simulink model "Resonator16_order_FIR"  (R2019a)
settings: Solver=FixedStepDiscrete  StartTime=0.0  StopTime=10  FixedStep=0.001  RelTol=1e-3
libraries: dspxfrm3 x2, simulink x1
settings Model: Creator=vardhah  LastModifiedBy=vardhah
settings DataIOCC: ReturnWorkspaceOutputs=off
settings DebuggingCC: ArithmeticOperatorsInVariantConditions=warning

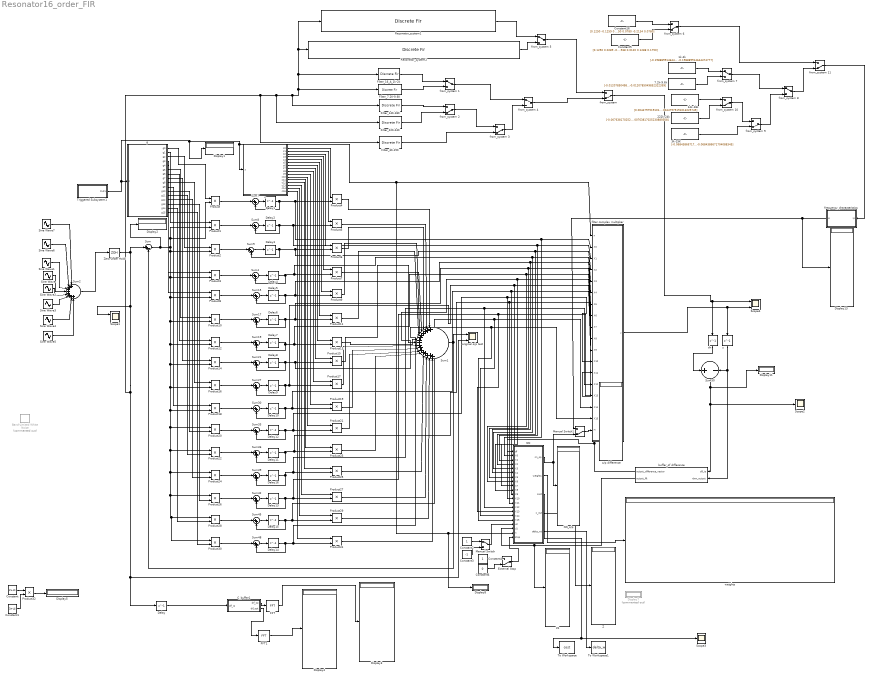
== system Resonator16_order_FIR ==
  "14k-18k " : Constant  Value=[0.00447975191013225745 0.0111493911810838543 0.0275893297063002849 -0.183954681451905411 0.0755136163583744469 0.0976817056268990125 -0.238475271342986128 0.121471156344241021 0.121471156344241021 -0.238475271342986128 0.0976817056268990125 0.0755136163583744469 -0.183954681451905411 0.0275893297063002849 0.0111493911810838543 0.00447975191013225745]  VectorParams1D=off
  1k-2k : Constant  Value=[-0.198889914644374777 0.0882189428518377339 0.0736891495871065116 0.0638368801789635787 0.0566372642221577294 0.0523172683654103132 0.0494565343907736044 0.048157521822162791 0.048157521822162791 0.0494565343907736044 0.0523172683654103132 0.0566372642221577294 0.0638368801789635787 0.0736891495871065116 0.0882189428518377339 -0.198889914644374777]  VectorParams1D=off
  222k-24k : Constant  Value=[-0.00763817025230889308 0.108944026972857946 -0.0989847012675625776 0.124240247797868963 -0.129657713018954679 0.114438069344974691 -0.0787108015776764036 0.0280491419731783154 0.0280491419731783154 -0.0787108015776764036 0.114438069344974691 -0.129657713018954679 0.124240247797868963 -0.0989847012675625776 0.108944026972857946 -0.00763817025230889308]  VectorParams1D=off
  3k-15K : Constant  Value=[-0.0684386671704088345 -0.0216035519389094557 -0.0869907772510868094 -0.0695372998678755599 0.0160068430386171648 -0.171506412844009415 -0.104404398490726372 0.48413102780480427 0.48413102780480427 -0.104404398490726372 -0.171506412844009415 0.0160068430386171648 -0.0695372998678755599 -0.0869907772510868094 -0.0216035519389094557 -0.0684386671704088345]  VectorParams1D=off
  "7.2k-9.6k " : Constant  Value=[-0.0120785049852322399 -0.0942455273574688279 0.0101245004695954266 0.125460404555770566 0.034165372769331126 -0.1614987160724079 -0.0984930555982914957 0.150982315564688691 0.150982315564688691 -0.0984930555982914957 -0.1614987160724079 0.034165372769331126 0.125460404555770566 0.0101245004695954266 -0.0942455273574688279 -0.0120785049852322399]  VectorParams1D=off
  Band-Limited White Noise : simulink/Sources/Band-Limited White Noise  Commented=on  Cov=[0.5]  Ts=0.000003  seed=[23341]
  C_buffer1 : MATLAB Function  TreatAsAtomicUnit=on
  Constant : Constant  Value=2+3i
  Constant1 : Constant  Value=3+4i
  Constant16 : Constant  Value=[0.1250 -0.1259 0 0.0375 0 0.0104 -0.0366 0.0104 0 0.0375 0 -0.1259 0.1250 0.0780 -0.2134 0.0780]  VectorParams1D=off
  Constant2 : Constant
  Constant3 : Constant  Value=-1
  Constant4 : Constant
  Constant5 : Constant  Value=[0.1250 0.0289 -0.0404 -0.0525 -0.0313 -0.0120 -0.0038 0.0018 0 -0.0289 -0.0846 -0.1243 -0.0938 0.0120 0.1288 0.1750]  VectorParams1D=off
  Constant6 : Constant  Value=0
  Delay{,1..16} (17 alike) : Delay  DelayLength=1  InitialCondition=0
  Display{1..5,8,11,13} (8 alike) : Display
  Display7 : Display  Commented=on
  External Stop : ManualSwitch  CurrentSetting=0
  FFT : dspxfrm3/FFT  FFTImplementation=Auto  CompMethod=Table lookup  TableOpt=NEW  TableOptActive=Speed  BitRevOrder=off  Normalize=on  InheritFFTLength=on  FFTLength=64  WrapInput=on  roundingMode=Floor  overflowMode=off  firstCoeffDataTypeStr=Inherit: Same word length as input  firstCoeffLastDataTypeStr=Inherit: Same word length as input  outputMin=[]  outputMax=[]
  FFT1 : dspxfrm3/FFT  FFTImplementation=Auto  CompMethod=Table lookup  TableOpt=NEW  TableOptActive=Speed  BitRevOrder=off  Normalize=on  InheritFFTLength=on  FFTLength=64  WrapInput=on  roundingMode=Floor  overflowMode=off  firstCoeffDataTypeStr=Inherit: Same word length as input  firstCoeffLastDataTypeStr=Inherit: Same word length as input  outputMin=[]  outputMax=[]
  Filter_14K-18K : DiscreteFir  Tag=BlockMethodSubSystem  Coefficients=[0.00447975191013225745 0.0111493911810838543 0.0275893297063002849 -0.183954681451905411 0.0755136163583744469 0.0976817056268990125 -0.238475271342986128 0.121471156344241021 0.121471156344241021 -0.238475271342986128 0.0976817056268990125 0.0755136163583744469 -0.183954681451905411 0.0275893297063002849 0.0111493911810838543 0.00447975191013225745]  InputProcessing=Columns as channels (frame based)
  Filter_16_A_1k-2k : DiscreteFir  Tag=BlockMethodSubSystem  Coefficients=[-0.198889914644374777 0.0882189428518377339 0.0736891495871065116 0.0638368801789635787 0.0566372642221577294 0.0523172683654103132 0.0494565343907736044 0.048157521822162791 0.048157521822162791 0.0494565343907736044 0.0523172683654103132 0.0566372642221577294 0.0638368801789635787 0.0736891495871065116 0.0882189428518377339 -0.198889914644374777]  InputProcessing=Columns as channels (frame based)
  Filter_22K-24K : DiscreteFir  Tag=BlockMethodSubSystem  Coefficients=[-0.00763817025230889308 0.108944026972857946 -0.0989847012675625776 0.124240247797868963 -0.129657713018954679 0.114438069344974691 -0.0787108015776764036 0.0280491419731783154 0.0280491419731783154 -0.0787108015776764036 0.114438069344974691 -0.129657713018954679 0.124240247797868963 -0.0989847012675625776 0.108944026972857946 -0.00763817025230889308]  InputProcessing=Columns as channels (frame based)
  Filter_3K-15K : DiscreteFir  Tag=BlockMethodSubSystem  Coefficients=[-0.0684386671704088345 -0.0216035519389094557 -0.0869907772510868094 -0.0695372998678755599 0.0160068430386171648 -0.171506412844009415 -0.104404398490726372 0.48413102780480427 0.48413102780480427 -0.104404398490726372 -0.171506412844009415 0.0160068430386171648 -0.0695372998678755599 -0.0869907772510868094 -0.0216035519389094557 -0.0684386671704088345]  InputProcessing=Columns as channels (frame based)
  "Filter_7.2K-9.6K " : DiscreteFir  Tag=BlockMethodSubSystem  Coefficients=[-0.0120785049852322399 -0.0942455273574688279 0.0101245004695954266 0.125460404555770566 0.034165372769331126 -0.1614987160724079 -0.0984930555982914957 0.150982315564688691 0.150982315564688691 -0.0984930555982914957 -0.1614987160724079 0.034165372769331126 0.125460404555770566 0.0101245004695954266 -0.0942455273574688279 -0.0120785049852322399]  InputProcessing=Columns as channels (frame based)
  Manual Switch : ManualSwitch
  Manual Switch1 : ManualSwitch  CurrentSetting=0  varsize=on
  NN : MATLAB Function  TreatAsAtomicUnit=on
  NN_o/p : Display
  Product{,1..32} (33 alike) : Product
  "Rezonator_system1 " : DiscreteFir  Tag=BlockMethodSubSystem  Coefficients=[0.1250 -0.1259 0 0.0375 0 0.0104 -0.0366 0.0104 0 0.0375 0 -0.1259 0.1250 0.0780 -0.2134 0.0780]  InputProcessing=Columns as channels (frame based)
  Rezonator_system2 : DiscreteFir  Tag=BlockMethodSubSystem  Coefficients=[0.1250 0.0289 -0.0404 -0.0525 -0.0313 -0.0120 -0.0038 0.0018 0 -0.0289 -0.0846 -0.1243 -0.0938 0.0120 0.1288 0.1750]  InputProcessing=Columns as channels (frame based)
  Scope1 : Scope  NumInputPorts=2
  Scope2 : Scope
  Scope3 : Scope
  Scope4 : Scope  NumInputPorts=2
  Sine Wave : Sin  Amplitude=0  Frequency=5000  SampleTime=0
  Sine Wave1 : Sin  Amplitude=0  Frequency=7000  SampleTime=0
  Sine Wave2 : Sin  Amplitude=0  Frequency=2000  SampleTime=0
  Sine Wave3 : Sin  Amplitude=0  Frequency=479  SampleTime=0
  Sine Wave4 : Sin  Amplitude=0  Frequency=100  SampleTime=0
  Sine Wave5 : Sin  Amplitude=3  Frequency=50  SampleTime=0
  Sine Wave6 : Sin  Amplitude=0  Frequency=11000  SampleTime=0
  Sine Wave7 : Sin  Amplitude=0  Frequency=17000  SampleTime=0
  Sum : Sum  Inputs=|+-
  Sum1 : Sum  Inputs=|++++++++++++++++
  Sum{4,7..9,15,17,19,21,27,30,33,36,39,42,45,48} (16 alike) : Sum  Inputs=|++
  Sum2 : Sum  Inputs=|++++++++
  Sum50 : Sum  Inputs=+-
  To Workspace : ToWorkspace  VariableName=cost  SampleTime=-1
      settings: Save2DSignal=2-D array (concatenate along first dimension)
  To Workspace1 : ToWorkspace  VariableName=delta_w  SampleTime=-1
      settings: Save2DSignal=2-D array (concatenate along first dimension)
  Triggered Subsystem1 : Subsystem  TreatAsAtomicUnit=on
  Z : Display
  Z1 : Display
  Zero-Order Hold : ZeroOrderHold  SampleTime=0.001
  buffer_of difference : MATLAB Function  TreatAsAtomicUnit=on
  c : MATLAB Function  TreatAsAtomicUnit=on
  dn : Delay  DelayLength=1  InitialCondition=0
  filter complex multiplier : MATLAB Function  TreatAsAtomicUnit=on
  frequency_characteristics : MATLAB Function  TreatAsAtomicUnit=on
  from_system {,2..3,6,9..11} (7 alike) : ManualSwitch  CurrentSetting=0
  from_system {1,4..5,7..8} (5 alike) : ManualSwitch
  g : MATLAB Function  TreatAsAtomicUnit=on
  o/p difference : Display
  "original o/p test " : Scope  NumInputPorts=2
  weights : Display
  y : Delay  DelayLength=1  InitialCondition=0
  wires:
  Delay1/1 -> filter complex multiplier/2(X0), NN/2(X0), Product4/2, Sum7/2
  c/1(c0) -> Product4/1
  c/2(c1) -> Product5/1
  c/3(c2) -> Product6/1
  c/4(c3) -> Product7/1
  Delay2/1 -> Sum8/2, filter complex multiplier/3(X1), NN/3(X1), Product5/2
  Delay3/1 -> NN/4(X2), filter complex multiplier/4(X2), Product6/2, Sum9/2
  Delay4/1 -> Sum4/2, NN/5(X3), filter complex multiplier/5(X3), Product7/2
  Sum1/1 -> "original o/p test "/1, Sum/2
  g/1(g0) -> Product/1
  g/2(g1) -> Product1/1
  g/3(g2) -> Product2/1
  g/4(g3) -> Product3/1
  Sum4/1 -> Delay4/1
  Sum9/1 -> Delay3/1
  Sum8/1 -> Delay2/1
  Sum7/1 -> Delay1/1
  Product4/1 -> Sum1/1
  Product5/1 -> Sum1/2
  Product6/1 -> Sum1/3
  Product7/1 -> Sum1/4
  Triggered Subsystem1/1(Out1) -> Display1/1, c/1(n), Display8/1, NN/20(n), filter complex multiplier/1(n), g/1(n)
  Sum/1 -> Display2/1, Product1/2, Product/2, Product2/2, Product10/2, Product12/2, Product14/2, Product16/2, Product30/1, Product28/1, Product26/1, Product24/1, Product22/1, Product20/1, Product18/2, Product8/2, Product3/2
  Product3/1 -> Sum4/1
  Product2/1 -> Sum9/1
  Product1/1 -> Sum8/1
  Product/1 -> Sum7/1
  Product8/1 -> Sum15/1
  Sum15/1 -> Delay5/1
  Delay5/1 -> filter complex multiplier/6(X4), NN/6(X4), Product9/2, Sum15/2
  Product10/1 -> Sum17/1
  Sum17/1 -> Delay6/1
  Delay6/1 -> filter complex multiplier/7(X5), NN/7(X5), Product11/2, Sum17/2
  Product12/1 -> Sum19/1
  Sum19/1 -> Delay7/1
  Delay7/1 -> filter complex multiplier/8(X6), NN/8(X6), Product13/2, Sum19/2
  Product14/1 -> Sum21/1
  Sum21/1 -> Delay8/1
  Delay8/1 -> filter complex multiplier/9(X7), NN/9(X7), Product15/2, Sum21/2
  g/5(g4) -> Product8/1
  g/6(g5) -> Product10/1
  g/7(g6) -> Product12/1
  g/8(g7) -> Product14/1
  c/5(c4) -> Product9/1
  c/6(c5) -> Product11/1
  c/7(c6) -> Product13/1
  c/8(c7) -> Product15/1
  Product9/1 -> Sum1/5
  Product11/1 -> Sum1/6
  Product13/1 -> Sum1/7
  Product15/1 -> Sum1/8
  Product16/1 -> Sum27/1
  Sum27/1 -> Delay9/1
  Delay9/1 -> Product17/2, filter complex multiplier/10(X8), NN/10(X8), Sum27/2
  Sum30/1 -> Delay10/1
  Delay10/1 -> filter complex multiplier/11(X9), NN/11(X9), Product19/2, Sum30/2
  Product18/1 -> Sum30/1
  Sum33/1 -> Delay12/1
  Delay12/1 -> NN/12(X10), filter complex multiplier/12(X10), Product21/2, Sum33/2
  Product22/1 -> Sum36/1
  Product20/1 -> Sum33/1
  Sum36/1 -> Delay11/1
  Sum39/1 -> Delay16/1
  Product26/1 -> Sum42/1
  Sum42/1 -> Delay13/1
  Delay16/1 -> filter complex multiplier/14(X12), NN/14(X12), Product25/2, Sum39/2
  Product24/1 -> Sum39/1
  Delay14/1 -> NN/17(X15), filter complex multiplier/17(X15), Product31/2, Sum48/2
  Sum45/1 -> Delay15/1
  Sum48/1 -> Delay14/1
  Product30/1 -> Sum48/1
  Product28/1 -> Sum45/1
  Delay15/1 -> NN/16(X14), filter complex multiplier/16(X14), Product29/2, Sum45/2
  c/9(c8) -> Product17/1
  c/10(c9) -> Product19/1
  c/11(c10) -> Product21/1
  c/12(c11) -> Product23/1
  c/13(c12) -> Product25/1
  c/14(c13) -> Product27/1
  c/15(c14) -> Product29/1
  c/16(c15) -> Product31/1
  g/9(g8) -> Product16/1
  g/10(g9) -> Product18/1
  g/11(g10) -> Product20/2
  g/12(g11) -> Product22/2
  g/13(g12) -> Product24/2
  g/14(g13) -> Product26/2
  g/15(g14) -> Product28/2
  g/16(g15) -> Product30/2
  Product17/1 -> Sum1/9
  Product19/1 -> Sum1/10
  Product21/1 -> Sum1/11
  Product23/1 -> Sum1/12
  Product25/1 -> Sum1/13
  Product27/1 -> Sum1/14
  Product29/1 -> Sum1/15
  Product31/1 -> Sum1/16
  filter complex multiplier/1(y) -> y/1, Scope4/2
  C_buffer1/1(dif_op) -> FFT/1
  FFT/1 -> Display3/1
  C_buffer1/2(dif_opt) -> FFT1/1
  FFT1/1 -> Display4/1
  Delay/1 -> C_buffer1/1(dif_ip)
  Zero-Order Hold/1 -> Sum/1, Delay/1, "original o/p test "/2, Filter_3K-15K/1, Filter_22K-24K/1, Filter_14K-18K/1, "Rezonator_system1 "/1, Rezonator_system2/1, Filter_16_A_1k-2k/1, "Filter_7.2K-9.6K "/1, Scope1/1
  "from_system "/1 -> dn/1, Scope4/1
  Filter_3K-15K/1 -> from_system 3/2
  from_system 2/1 -> from_system 3/1
  Filter_22K-24K/1 -> from_system 2/2
  Filter_14K-18K/1 -> from_system 2/1
  "Filter_7.2K-9.6K "/1 -> from_system 1/2
  Filter_16_A_1k-2k/1 -> from_system 1/1
  from_system 3/1 -> from_system 4/2
  from_system 1/1 -> from_system 4/1
  from_system 4/1 -> "from_system "/2
  "Rezonator_system1 "/1 -> from_system 5/1
  Rezonator_system2/1 -> from_system 5/2
  from_system 5/1 -> "from_system "/1
  Constant16/1 -> from_system 6/1
  Constant5/1 -> from_system 6/2
  1k-2k/1 -> from_system 7/1
  "7.2k-9.6k "/1 -> from_system 7/2
  "14k-18k "/1 -> from_system 10/1
  222k-24k/1 -> from_system 10/2
  3k-15K/1 -> from_system 9/2
  from_system 10/1 -> from_system 9/1
  from_system 9/1 -> from_system 8/2
  from_system 7/1 -> from_system 8/1
  from_system 6/1 -> from_system 11/1
  from_system 8/1 -> from_system 11/2
  Constant/1 -> Product32/1
  Constant1/1 -> Product32/2
  Product32/1 -> Display5/1
  Sine Wave7/1 -> Sum2/1
  Sine Wave6/1 -> Sum2/2
  Sine Wave1/1 -> Sum2/3
  Sine Wave/1 -> Sum2/4
  Sine Wave2/1 -> Sum2/5
  Sine Wave3/1 -> Sum2/6
  Sine Wave4/1 -> Sum2/7
  Sine Wave5/1 -> Sum2/8
  Sum2/1 -> Zero-Order Hold/1
  dn/1 -> Sum50/1
  Sum50/1 -> Display11/1, buffer_of difference/1(dif_ip), Scope2/1
  Delay11/1 -> NN/13(X11), filter complex multiplier/13(X11), Product23/2, Sum36/2
  Delay13/1 -> NN/15(X13), filter complex multiplier/15(X13), Product27/2, Sum42/2
  Manual Switch/1 -> NN/18(u2)
  Constant2/1 -> Manual Switch/1
  Constant3/1 -> Manual Switch/2
  NN/2(weights) -> weights/1
  buffer_of difference/1(output_difference_vector) -> o/p difference/1, NN/1(df)
  NN/3(cost) -> Scope3/1, To Workspace/1
  NN/1(nn_op) -> NN_o/p/1, Manual Switch1/2
  from_system 11/1 -> frequency_characteristics/1(ip)
  Manual Switch1/1 -> filter complex multiplier/18(H)
  frequency_characteristics/1(H) -> Display13/1, Manual Switch1/1
  NN/4(z_out) -> Z/1
  NN/5(delta_wt) -> To Workspace1/1
  External Stop/1 -> NN/21(stop)
  Constant4/1 -> External Stop/1
  Constant6/1 -> External Stop/2
  y/1 -> Sum50/2, buffer_of difference/2(rbnn_output)
  buffer_of difference/2(output_fft) -> Z1/1, NN/19(u1)

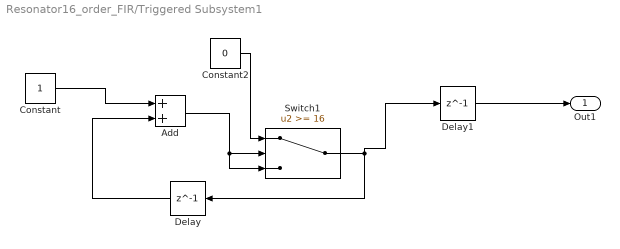
== system Resonator16_order_FIR/Triggered Subsystem1 ==
  Add : Sum
  Constant : Constant
  Constant2 : Constant  Value=0
  Delay : Delay  DelayLength=1  InitialCondition=0
  Delay1 : Delay  DelayLength=1  InitialCondition=0
  Switch1 : Switch  Threshold=16
  Out1 : Outport
  wires:
  Constant2/1 -> Switch1/1
  Constant/1 -> Add/1
  Switch1/1 -> Delay1/1, Delay/1
  Delay/1 -> Add/2
  Add/1 -> Switch1/3, Switch1/2
  Delay1/1 -> Out1/1

== matlab function Resonator16_order_FIR/c ==
  data: n input; c0 output; c1 output; c2 output; c3 output; c4 output; c5 output; c6 output; c7 output; c8 output; c9 output; c10 output; c11 output; c12 output; c13 output; c14 output; c15 output
function [c0,c1,c2,c3,c4,c5,c6,c7,c8,c9,c10,c11,c12,c13,c14,c15]  = fcn(n)
N=16;


c0=exp(1i*2*(pi/N)*0*n) ;    
c1=exp(1i*2*(pi/N)*1*n) ; 
c2=exp(1i*2*(pi/N)*2*n); 
c3=exp(1i*2*(pi/N)*3*n) ;
c4=exp(1i*2*(pi/N)*4*n) ;    
c5=exp(1i*2*(pi/N)*5*n); 
c6=exp(1i*2*(pi/N)*6*n); 
c7=exp(1i*2*(pi/N)*7*n); 
c8=exp(1i*2*(pi/N)*8*n) ;    
c9=exp(1i*2*(pi/N)*9*n); 
c10=exp(1i*2*(pi/N)*10*n); 
c11=exp(1i*2*(pi/N)*11*n);
c12=exp(1i*2*(pi/N)*12*n) ;    
c13=exp(1i*2*(pi/N)*13*n); 
c14=exp(1i*2*(pi/N)*14*n); 
c15=exp(1i*2*(pi/N)*15*n);

== matlab function Resonator16_order_FIR/g ==
  data: n input; g0 output; g1 output; g2 output; g3 output; g4 output; g5 output; g6 output; g7 output; g8 output; g9 output; g10 output; g11 output; g12 output; g13 output; g14 output; g15 output
function [g0,g1,g2,g3,g4,g5,g6,g7,g8,g9,g10,g11,g12,g13,g14,g15]  = fcn(n)
N=16;


g0=1/N*exp(-1i*2*(pi/N)*0*n) ;    
g1=1/N*exp(-1i*2*(pi/N)*1*n); 
g2=1/N*exp(-1i*2*(pi/N)*2*n); 
g3=1/N*exp(-1i*2*(pi/N)*3*n);
g4=1/N*exp(-1i*2*(pi/N)*4*n) ;    
g5=1/N*exp(-1i*2*(pi/N)*5*n); 
g6=1/N*exp(-1i*2*(pi/N)*6*n); 
g7=1/N*exp(-1i*2*(pi/N)*7*n); 
g8=1/N*exp(-1i*2*(pi/N)*8*n);    
g9=1/N*exp(-1i*2*(pi/N)*9*n); 
g10=1/N*exp(-1i*2*(pi/N)*10*n); 
g11=1/N*exp(-1i*2*(pi/N)*11*n);
g12=1/N*exp(-1i*2*(pi/N)*12*n) ;    
g13=1/N*exp(-1i*2*(pi/N)*13*n); 
g14=1/N*exp(-1i*2*(pi/N)*14*n); 
g15=1/N*exp(-1i*2*(pi/N)*15*n);

== matlab function Resonator16_order_FIR/filter complex multiplier ==
  data: n input; X0 input; y output; X1 input; X2 input; X3 input; X4 input; X5 input; X6 input; X7 input; X8 input; X9 input; X10 input; X11 input; X12 input; X13 input; X14 input; X15 input; H input size=16
    function y   = fcn(n,X0,X1,X2,X3,X4,X5,X6,X7,X8,X9,X10,X11,X12,X13,X14,X15,H)

NN=transpose(H);

F=transpose([real(X0) 2*(real(X1)*cos(pi*1*n/8)-imag(X1)*sin(pi*1*n/8)) 2*(real(X2)*cos(pi*2*n/8)-imag(X2)*sin(pi*2*n/8)) 2*(real(X3)*cos(pi*3*n/8)-imag(X3)*sin(pi*3*n/8)) 2*(real(X4)*cos(pi*4*n/8)-imag(X4)*sin(pi*4*n/8)) 2*(real(X5)*cos(pi*5*n/8)-imag(X5)*sin(pi*5*n/8)) 2*(real(X6)*cos(pi*6*n/8)-imag(X6)*sin(pi*6*n/8)) 2*(real(X7)*cos(pi*7*n/8)-imag(X7)*sin(pi*7*n/8)) -1^n*real(X8) -2*(imag(X9)*cos(pi*9*n/8)+real(X9)*sin(pi*9*n/8)) -2*(imag(X10)*cos(pi*10*n/8)+real(X10)*sin(pi*10*n/8)) -2*(imag(X11)*cos(pi*11*n/8)+real(X11)*sin(pi*11*n/8)) -2*(imag(X12)*cos(pi*12*n/8)+real(X12)*sin(pi*12*n/8)) -2*(imag(X13)*cos(pi*13*n/8)+real(X13)*sin(pi*13*n/8)) -2*(imag(X14)*cos(pi*14*n/8)+real(X14)*sin(pi*14*n/8)) -2*(imag(X15)*cos(pi*15*n/8)+real(X15)*sin(pi*15*n/8))]); 

y= NN*F; 


end

== matlab function Resonator16_order_FIR/buffer_of difference ==
  data: dif_ip input; output_difference_vector output size=[1,16]; rbnn_output input; output_fft output size=[1,16]
function [output_difference_vector,output_fft] = difBuffer(dif_ip,rbnn_output)                      

 sz=16;                    % size of the dft 
 
 persistent a;
 if isempty(a)
  a= zeros(1,sz);
 end
 a= circshift(a,1);
 a(1)=dif_ip;
 output_difference_vector=a; 

 persistent b;
 if isempty(b)
  b= zeros(1,sz);
 end
 b= circshift(b,1);
 b(1)=rbnn_output;
 output_fft=1/sz*fft(b); 
 
end

== matlab function Resonator16_order_FIR/C_buffer1 ==
  data: dif_ip input; dif_op output size=16; dif_opt output size=16
function [dif_op,dif_opt]  = difBuffer(dif_ip)                      
 
 persistent d0 d1 d2 d3 d4 d5 d6 d7 d8 d9 d10 d11 d12 d13 d14 d15;  
  
 if isempty(d0)
        d0 = 0i;
 end
 if isempty(d1)
        d1 = 0i;
 end
 if isempty(d2)
        d2 = 0i;
 end 
 if isempty(d3)
        d3 = 0i;
 end
 if isempty(d4)
        d4 = 0i;
 end
 if isempty(d5)
        d5 = 0i;
 end
 if isempty(d6)
        d6 = 0i;
 end
 if isempty(d7)
        d7 = 0i;
 end
 if isempty(d8)
        d8 = 0i;
 end
 if isempty(d9)
        d9 = 0i;
 end
 if isempty(d10)
        d10 = 0i;
 end
 if isempty(d11)
        d11 = 0i;
 end
 if isempty(d12)
        d12 = 0i;
 end
 if isempty(d13)
     d13 = 0i;end
 if isempty(d14)
     d14 = 0i;end
 if isempty(d15)
     d15 = 0i;
 end
 
 
 d15=d14;
 d14=d13;
 d13=d12;
 d12=d11;
 d11=d10;
 d10=d9;
 d9=d8;
 d8=d7;
 d7=d6;
 d6=d5;
 d5=d4;
 d4=d3; 
 d3=d2;
 d2=d1;
 d1=d0;
 d0=dif_ip;
 dif_op=[d0 d1 d2 d3 d4 d5 d6 d7 d8 d9 d10 d11 d12 d13 d14 d15]';
 dif_opt=[d15 d14 d13 d12 d11 d10 d9 d8 d7 d6 d5 d4 d3 d2 d1 d0]';

== matlab function Resonator16_order_FIR/NN ==
  settings: sampleTime=0.01
  data: nn_op output size=16; df input size=[1,16]; X0 input; X1 input; X2 input; X3 input; X4 input; X5 input; X6 input; X7 input; X8 input; X9 input; X10 input; X11 input; X12 input; X13 input; X14 input; X15 input; u2 input; u1 input size=[1,16]; n input; weights output; cost output; z_out output; delta_wt output; stop input
function [nn_op,weights,cost,z_out,delta_wt]  = NN(df,X0,X1,X2,X3,X4,X5,X6,X7,X8,X9,X10,X11,X12,X13,X14,X15,u2,u1,n,stop)

persistent w1;
persistent vy;
persistent g;
persistent itr;
persistent J;
persistent del_w;
persistent mult;
persistent memory_alloc_flag;


%layer declaration
input_layer = 17; 
layer_1=16;

if isempty(memory_alloc_flag)
        memory_alloc_flag = 0; 
end
if isempty(mult)
       mult=zeros(layer_1,layer_1*input_layer); 
end
if memory_alloc_flag==0
 %write memory allocation for looped code here.. 
 mult=[];
  for itr =1:layer_1
   mult=[mult;[zeros(1,(itr-1)*input_layer) ones(1,input_layer) zeros(1,(input_layer-itr-1)*input_layer)]];
 end
 memory_alloc_flag=1;
end

if isempty(del_w)
    del_w=zeros(1,272);
end

if isempty(itr)
    itr=0;
end
if isempty(J)
    J=0;
end

%gradient initialisation
if isempty(g)
    g= zeros(16,272);
   %g= rand(16,272);   
end


%prestored Vy matrix
if isempty(vy)
    vy=[0.0625000000000000,0.0625000000000000,0.0625000000000000,0.0625000000000000,0.0625000000000000,0.0625000000000000,0.0625000000000000,0.0625000000000000,0.0625000000000000,0.0625000000000000,0.0625000000000000,0.0625000000000000,0.0625000000000000,0.0625000000000000,0.0625000000000000,0.0625000000000000;0.0577424707819554,0.0441941738241592,0.0239177145228181,-1.14810637420064e-17,-0.0239177145228181,-0.0441941738241592,-0.0577424707819554,-0.0625000000000000,-0.0577424707819554,-0.0441941738241592,-0.0239177145228181,3.82702124733548e-18,0.0239177145228181,0.0441941738241592,0.0577424707819554,0.0625000000000000;0.0441941738241592,-2.67891487313484e-17,-0.0441941738241592,-0.0625000000000000,-0.0441941738241592,1.91351062366774e-17,0.0441941738241592,0.0625000000000000,0.0441941738241592,-1.14810637420064e-17,-0.0441941738241592,-0.0625000000000000,-0.0441941738241592,3.82702124733548e-18,0.0441941738241592,0.0625000000000000;0.0239177145228179,-0.0441941738241592,-0.0577424707819554,3.44431912260193e-17,0.0577424707819555,0.0441941738241592,-0.0239177145228182,-0.0625000000000000,-0.0239177145228181,0.0441941738241592,0.0577424707819554,-1.14810637420064e-17,-0.0577424707819554,-0.0441941738241592,0.0239177145228181,0.0625000000000000;-1.68427621172548e-16,-0.0625000000000000,-6.12710262471544e-17,0.0625000000000000,-1.53119536183206e-16,-0.0625000000000000,3.44431912260193e-17,0.0625000000000000,-2.67891487313484e-17,-0.0625000000000000,1.91351062366774e-17,0.0625000000000000,-1.14810637420064e-17,-0.0625000000000000,3.82702124733548e-18,0.0625000000000000;-0.0239177145228182,-0.0441941738241591,0.0577424707819554,-1.68427621172548e-16,-0.0577424707819554,0.0441941738241592,0.0239177145228181,-0.0625000000000000,0.0239177145228182,0.0441941738241592,-0.0577424707819554,1.91351062366774e-17,0.0577424707819554,-0.0441941738241592,-0.0239177145228181,0.0625000000000000;-0.0441941738241596,-3.06548562684706e-17,0.0441941738241593,-0.0625000000000000,0.0441941738241594,-1.68427621172548e-16,-0.0441941738241592,0.0625000000000000,-0.0441941738241592,3.44431912260193e-17,0.0441941738241592,-0.0625000000000000,0.0441941738241592,-1.14810637420064e-17,-0.0441941738241592,0.0625000000000000;-0.0577424707819556,0.0441941738241594,-0.0239177145228178,-3.06548562684706e-17,0.0239177145228179,-0.0441941738241591,0.0577424707819554,-0.0625000000000000,0.0577424707819555,-0.0441941738241592,0.0239177145228182,-2.67891487313484e-17,-0.0239177145228181,0.0441941738241592,-0.0577424707819554,0.0625000000000000;-0.0625000000000000,0.0625000000000000,-0.0625000000000000,0.0625000000000000,-0.0625000000000000,0.0625000000000000,-0.0625000000000000,0.0625000000000000,-0.0625000000000000,0.0625000000000000,-0.0625000000000000,0.0625000000000000,-0.0625000000000000,0.0625000000000000,-0.0625000000000000,0.0625000000000000;-0.0239177145228184,0.0441941738241592,-0.0577424707819555,0.0625000000000000,-0.0577424707819553,0.0441941738241592,-0.0239177145228180,-6.88863824520386e-17,0.0239177145228181,-0.0441941738241593,0.0577424707819554,-0.0625000000000000,0.0577424707819554,-0.0441941738241592,0.0239177145228181,0;-0.0441941738241594,0.0625000000000000,-0.0441941738241593,-3.36855242345096e-16,0.0441941738241595,-0.0625000000000000,0.0441941738241592,7.65404249467096e-17,-0.0441941738241593,0.0625000000000000,-0.0441941738241592,-3.82702124733548e-17,0.0441941738241593,-0.0625000000000000,0.0441941738241592,0;-0.0577424707819556,0.0441941738241592,0.0239177145228178,-0.0625000000000000,0.0239177145228177,0.0441941738241592,-0.0577424707819555,-3.06239072366412e-16,0.0577424707819554,-0.0441941738241592,-0.0239177145228181,0.0625000000000000,-0.0239177145228181,-0.0441941738241593,0.0577424707819554,0;-0.0625000000000000,6.13097125369412e-17,0.0625000000000000,1.37772764904077e-16,-0.0625000000000000,-3.36855242345096e-16,0.0625000000000000,9.18485099360515e-17,-0.0625000000000000,-6.88863824520386e-17,0.0625000000000000,4.59242549680257e-17,-0.0625000000000000,-2.29621274840129e-17,0.0625000000000000,0;-0.0577424707819553,-0.0441941738241594,0.0239177145228181,0.0625000000000000,0.0239177145228186,-0.0441941738241590,-0.0577424707819555,1.22542052494309e-16,0.0577424707819554,0.0441941738241593,-0.0239177145228180,-0.0625000000000000,-0.0239177145228182,0.0441941738241592,0.0577424707819554,0;-0.0441941738241587,-0.0625000000000000,-0.0441941738241588,6.13097125369412e-17,0.0441941738241588,0.0625000000000000,0.0441941738241592,1.07156594925393e-16,-0.0441941738241590,-0.0625000000000000,-0.0441941738241593,-5.35782974626967e-17,0.0441941738241592,0.0625000000000000,0.0441941738241592,0;-0.0239177145228178,-0.0441941738241593,-0.0577424707819556,-0.0625000000000000,-0.0577424707819556,-0.0441941738241594,-0.0239177145228184,-3.36855242345096e-16,0.0239177145228181,0.0441941738241592,0.0577424707819554,0.0625000000000000,0.0577424707819554,0.0441941738241593,0.0239177145228182,0;0,0,0,0,0,0,0,0,0,0,0,0,0,0,0,0];
end



%input initialisation
x_in = [real(u1(1)) real(u1(2)) real(u1(3)) real(u1(4)) real(u1(5)) real(u1(6)) real(u1(7)) real(u1(8)) real(u1(9)) imag(u1(1)) imag(u1(2)) imag(u1(3)) imag(u1(4)) imag(u1(5)) imag(u1(6)) imag(u1(7))];

%parameter intialisation 
v=transpose([x_in u2]);
if isempty(w1)
       w1=randn(input_layer,layer_1)*0.1;
end
alpha = 0.9;

F=transpose([real(X0) 2*(real(X1)*cos(pi*1*n/8)-imag(X1)*sin(pi*1*n/8)) 2*(real(X2)*cos(pi*2*n/8)-imag(X2)*sin(pi*2*n/8)) 2*(real(X3)*cos(pi*3*n/8)-imag(X3)*sin(pi*3*n/8)) 2*(real(X4)*cos(pi*4*n/8)-imag(X4)*sin(pi*4*n/8)) 2*(real(X5)*cos(pi*5*n/8)-imag(X5)*sin(pi*5*n/8)) 2*(real(X6)*cos(pi*6*n/8)-imag(X6)*sin(pi*6*n/8)) 2*(real(X7)*cos(pi*7*n/8)-imag(X7)*sin(pi*7*n/8)) -1^n*real(X8) -2*(imag(X9)*cos(pi*9*n/8)+real(X9)*sin(pi*9*n/8)) -2*(imag(X10)*cos(pi*10*n/8)+real(X10)*sin(pi*10*n/8)) -2*(imag(X11)*cos(pi*11*n/8)+real(X11)*sin(pi*11*n/8)) -2*(imag(X12)*cos(pi*12*n/8)+real(X12)*sin(pi*12*n/8)) -2*(imag(X13)*cos(pi*13*n/8)+real(X13)*sin(pi*13*n/8)) -2*(imag(X14)*cos(pi*14*n/8)+real(X14)*sin(pi*14*n/8)) -2*(imag(X15)*cos(pi*15*n/8)+real(X15)*sin(pi*15*n/8))]); 
%u_out=v;


%forward propogation
z=w1'*v ;
z_out=z;
a=(1./(1+exp(-z)));
an=(a-0.5);

%calculation of Nv:
dz_a=a.*(1-a);                  
Nv=w1'.* repmat(dz_a,1, size(w1,1));

%calculation of aD
aD=transpose(F)*Nv*vy;
A=[aD;eye(15) zeros(15,1)];
B=[transpose(F) ; zeros(15,16)];   
dw1=v*transpose(dz_a);

%added to vectorise the implementation
Expanded_dw1=repmat(transpose(dw1),1,size(dw1,2));
Nw=Expanded_dw1.*mult; 
g=A*g+B*Nw;


%Unvectorised implementation of above vectorised implementation:
%{
k=0; 
for j=1:16
    for i= 1:17 
        l=k+i;
        nw=zeros(16,1);
        nw(j,1)=dw1(i,j);
        g(:,l)=A*g(:,l)+B*nw;
    end
    k=l;
end
%}

if n==15 && stop==0
    del_w =alpha*df*1*g/16 ;
    del_w_reshaped= reshape(del_w,[17,16]);
    w1=w1+ del_w_reshaped;
    itr=itr+1;
    J= 1/32*sum(df.^2,'all');
end
cost=J;
delta_wt=del_w;
weights=w1;


nn_op=an;


end

== matlab function Resonator16_order_FIR/frequency_characteristics ==
  data: ip input; H output size=16
function H   = freq_character(ip)                      
dif_ip=fft(ip); 
H= [real(dif_ip(1)); real(dif_ip(2)); real(dif_ip(3));
real(dif_ip(4));
real(dif_ip(5));
real(dif_ip(6));
real(dif_ip(7));
real(dif_ip(8));
real(dif_ip(9));
imag(dif_ip(2));
imag(dif_ip(3));
imag(dif_ip(4));
imag(dif_ip(5));
imag(dif_ip(6));
imag(dif_ip(7));
imag(dif_ip(8));];
